simulink model "lec_11_train"  (R2021a)
settings: Solver=VariableStepAuto  StartTime=0.0  StopTime=1000  RelTol=1e-3
values from neighbouring files (symbols this model uses):
  g = 9.8    [lec_12_train_constant.m]    (also in lec_7_1_ss.m = 9.81)
  k = 20    [lec1_1_pid.m]    (also in lec_12_train_constant.m = 1; lec_7_1_ss.m = 0.0001)
  M1 = 1    [lec_12_train_constant.m]
  M2 = 0.5    [lec_12_train_constant.m]
  mu = 0.02    [lec_12_train_constant.m]
settings Model: Creator=d2h10s  LastModifiedBy=d2h10s

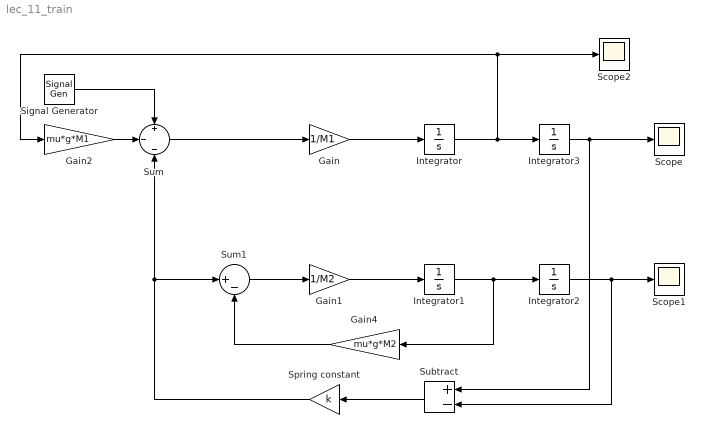
== system lec_11_train ==
  Gain : Gain  Gain=1/M1
  Gain1 : Gain  Gain=1/M2
  Gain2 : Gain  Gain=mu*g*M1
  Gain4 : Gain  Gain=mu*g*M2
  Integrator{,1..3} (4 alike) : Integrator
  Scope : Scope
  Scope1 : Scope
  Scope2 : Scope
  Signal Generator : SignalGenerator  WaveForm=square  Amplitude=-1  Frequency=0.001
  Spring constant : Gain  Gain=k
  Subtract : Sum  Inputs=+-
  Sum : Sum  Inputs=+|-|-
  Sum1 : Sum  Inputs=|+-
  wires:
  Sum/1 -> Gain/1
  Sum1/1 -> Gain1/1
  Gain/1 -> Integrator/1
  Gain1/1 -> Integrator1/1
  Integrator1/1 -> Gain4/1, Integrator2/1
  Integrator3/1 -> Subtract/1, Scope/1
  Integrator2/1 -> Subtract/2, Scope1/1
  Signal Generator/1 -> Sum/1
  Gain2/1 -> Sum/2
  Subtract/1 -> Spring constant/1
  Spring constant/1 -> Sum/3, Sum1/1
  Gain4/1 -> Sum1/2
  Integrator/1 -> Scope2/1, Gain2/1, Integrator3/1
